simulink model "mchp_acim_dsPIC33A"  (R2025b)
settings: Solver=FixedStepDiscrete  StartTime=0.0  StopTime=25  FixedStep=Ts  RelTol=1e-3  EnableMultiTasking=on
values from neighbouring files (symbols this model uses):
  dataType = 'single'    [mchp_acim_foc_dsPIC33A_data.m]
  PWM_frequency = 20e3    (= 20000)    [mchp_acim_foc_dsPIC33A_data.m]
  PWM_frequency_mc = PWM_frequency    (= 20000)    [mchp_acim_foc_dsPIC33A_data.m]
  SpeedFilterCutoff = 40    [mchp_acim_foc_dsPIC33A_data.m]
  Ts = T_pwm    (= 5e-05)    [mchp_acim_foc_dsPIC33A_data.m]
  Ts_mc = T_pwm_mc    (= 5e-05)    [mchp_acim_foc_dsPIC33A_data.m]
  Ts_motor = T_pwm_mc    (= 5e-05)    [mchp_acim_foc_dsPIC33A_data.m]
  Ts_serialIn = 100e-3    (= 0.1)    [mchp_acim_foc_dsPIC33A_data.m]
undefined symbols (not defined in the file or in its folder): A0, A4, acim, ADC, appState, B0, C10, C11, C6, C7, C8, CS_param, D11, D12, DiscIntNeverNeededParam, estim_pll, estim_qei, inverter, Max, MaxPer, ms, NumBits1, NumBits2, P1, P17, P20, P39, P40, P41, P43, P44, P60, P61, PI_params_SI, Pin, PWM4_Trg1, Resol, s, target, us, VmaxPhase
libraries: simulink x47, MCHP_Blockset x24, mcbcontrolslib x5, mcbeeMathTransformLib x4, slpidlib x4, svdutilitieslib x1, autolibim x1, mcbplantlib x1
(part 1 of 6)
settings Model: ExtModeEnableFloating=off  ExtModeTrigDuration=20  VariantFading=off  Creator=I50990  LastModifiedBy=I73849
settings SolverCC: AlgebraicLoopSolver=TrustRegion
settings OptimizationCC: DefaultParameterBehavior=Inlined  DefaultUnderspecifiedDataType=single  InlineInvariantSignals=on  EnhancedBackFolding=on  BooleansAsBitfields=on  PassReuseOutputArgsAs=Individual arguments  ZeroExternalMemoryAtStartup=off  ZeroInternalMemoryAtStartup=off  OptimizeBlockOrder=speed  DifferentSizesBufferReuse=on  EfficientTunableParamExpr=on
settings DebuggingCC: MultiTaskDSMMsg=none  MultiTaskCondExecSysMsg=none  MultiTaskRateTransMsg=warning  ParameterTunabilityLossMsg=error  ArithmeticOperatorsInVariantConditions=warning
settings HardwareCC: ProdBitPerPointer=32.0  ProdBitPerSizeT=32.0  ProdBitPerPtrDiffT=32.0  ProdLargestAtomicInteger=Long  ProdWordSize=32.0  ProdLongLongMode=on  ProdHWDeviceType=Generic->Custom
settings ModelReferenceCC: ModelReferenceNumInstancesAllowed=Single
settings SFSimCC: MATLABDynamicMemAlloc=off  CustomCodeUndefinedFunction=UseInterfaceOnly
settings RTWCC: SystemTargetFile=MCHP_dsPIC33A_noTMF_stf.tlc  TLCOptions="-aExtModeXCPClassicInterface=0  -aCreateExtModeTypes=1 -aExtModeXCPSimulationTimeInTicks=1"  TemplateMakefile=MCHP_dsPIC33A.tmf  Toolchain=MPLAB XC-DSC - v3.31 for dsPIC DSCs (Microchip)  BuildConfiguration=Specify  GPUComputeCapability=3.5  Description=Microchip Embedded Target dsPIC33A no TMF (real-time)
settings CodeAppCC: ForceParamTrailComments=on  IgnoreCustomStorageClasses=off  MaxIdLength=255.0  OperatorAnnotations=on  SimulinkDataObjDesc=on  SFDataObjDesc=on  InsertBlockDesc=on
settings STFCustomTargetCC: SystemTargetFile=MCHP_dsPIC33A_noTMF_stf.tlc  TargetLangStandard=C99 (ISO)  MultiwordLength=256.0  ConcurrentExecutionCompliant=off  CombineOutputUpdateFcns=on  CombineSignalStateStructs=on  SuppressErrorStatus=on  ERTCustomFileBanners=on  SupportContinuousTime=off  RemoveResetFunc=on  MATLABClassNameForMDSCustomization=Simulink.SoftwareTarget.ERTCustomization  GRTInterface=off  UseToolchainInfoCompliant=on  AssemblyListing=off  LINKER_SCRIPT=p33AK128MC106.gld  OPTIM_GCC=-O2 -mno-eds-warn -mconst-in-data -mlarge-code -mlarge-data -mlarge-scalar -mlarge-aggregate -g -Wa,--reorder  GCC1=xc-dsc-gcc.exe  RTWGenSettings_txt="s.RefMasterBlk='mchp_acim_dsPIC33A/MCHV-230VAC-1.5kW Development Board dsPIC33AK128MC106 MC DIM/Microchip Master';s.ChipIdN='[33  128  106]';s.ChipIdL1='AK';s.ChipIdL2='MC';s.ChipIdL3=' ';s.arch3='33A';s.ChipId='33AK128MC106';s.Arch='8';s.bitFieldsSFR='3';s.ChipRAM='16384';s.ChipRAM_XBegin='16384';s.ChipRAM_dma='[-1 -1]';s.FuseConfigTxt='#pragma config FWDT_WDTEN = SW\\\\n#pragma config FICD_JTAGEN = OFF\\\\n';s.TimeStep_Timer='-1';s.TimeStep_SyncADC='1';s.ADPCFG='0';s.ANSEL_Exist='1';s.ANSEL='[-1 -1 -1 -1 -1 -1 -1 -1 -1 -1 -1]';s.TRIS='[65535  65535  64990  65503     -1     -1     -1     -1     -1     -1     -1     -1     -1     -1     -1     -1     -1     -1     -1     -1     -1     -1     -1     -1     -1     -1     -1     -1     -1     -1     -1     -1     -1     -1     -1     -1     -1     -1     -1     -1     -1     -1     -1     -1     -1     -1     -1     -1     -1     -1     -1     -1     -1     -1     -1     -1     -1]';s.RPOR='[-1         -1         -1         -1         -1         -1         -1         -1         -1         -1     589824         -1         -1         -1  184549376         -1         -1         -1         -1         -1]';s.RPINR='[-1       -1       -1       -1       -1       -1       -1    10279       -1  3997740       -1       -1       -1       -1       -1       -1       -1       -1       -1       -1       -1       -1]';s.LATSET='[-1 -1 -1 -1 -1 -1 -1 -1 -1 -1 -1 -1 -1 -1 -1 -1 -1 -1 -1 -1 -1 -1 -1 -1 -1 -1 -1 -1 -1 -1 -1 -1 -1 -1 -1 -1 -1 -1 -1 -1 -1 -1 -1 -1 -1 -1 -1 -1 -1 -1 -1 -1 -1 -1 -1 -1 -1]';s.LATCLR='[-1 -1 -1 -1 -1 -1 -1 -1 -1 -1 -1 -1 -1 -1 -1 -1 -1 -1 -1 -1 -1 -1 -1 -1 -1 -1 -1 -1 -1 -1 -1 -1 -1 -1 -1 -1 -1 -1 -1 -1 -1 -1 -1 -1 -1 -1 -1 -1 -1 -1 -1 -1 -1 -1 -1 -1 -1]';s.ODC='[-1 -1 -1 -1 -1 -1 -1 -1 -1 -1 -1 -1 -1 -1 -1 -1 -1 -1 -1 -1 -1 -1 -1 -1 -1 -1 -1 -1 -1 -1 -1 -1 -1 -1 -1 -1 -1 -1 -1 -1 -1 -1 -1 -1 -1 -1 -1 -1 -1 -1 -1 -1 -1 -1 -1 -1 -1]';s.CNPU='[-1 -1 -1 -1 -1 -1 -1 -1 -1 -1 -1 -1 -1 -1 -1 -1 -1 -1 -1 -1 -1 -1 -1 -1 -1 -1 -1 -1 -1 -1 -1 -1 -1 -1 -1 -1 -1 -1 -1 -1 -1 -1 -1 -1 -1 -1 -1 -1 -1 -1 -1 -1 -1 -1 -1 -1 -1]';s.CNPD='[-1 -1 -1 -1 -1 -1 -1 -1 -1 -1 -1 -1 -1 -1 -1 -1 -1 -1 -1 -1 -1 -1 -1 -1 -1 -1 -1 -1 -1 -1 -1 -1 -1 -1 -1 -1 -1 -1 -1 -1 -1 -1 -1 -1 -1 -1 -1 -1 -1 -1 -1 -1 -1 -1 -1 -1 -1]';s.PortConfigTxt=' ';s.CLKDIV='0';s.PLLFBD='-1';s.PLLDIV='16815713';s.QUARTZ='8000000';s.SWITCH_OSC='16386';s.PLLRNG='-1';s.MASTER_BusyFlag='-1';s.POWERSAVE='0';s.MIPS='200000000';s.FLASH_ECC='0';s.PBxDIV='[-1]';s.CLKx_INTDIV='[-1 -1 -1 -1  0  1  0  0  0 -1 -1  0 -1]';s.CLKx_FRACDIV='[-1   -1   -1   -1    0  256    0    0    0   -1   -1    0   -1]';s.AN_type2='1';s.ACLKCON_reg='-1';s.nTIMERS='1';s.nSCCP='4';s.DOS_04094_cpu_33a_v1_dspic33a='1';s.DOS_04436_perseus_dspic33a='1';s.DOS_04928_gpio_ports_upb_v2_dspic33a='1';s.DOS_02672_math_progcrc_upb_v1_dspic33a='1';s.DOS_04993_sec_32bit_cp_upb_v1_dspic33a='1';s.DOS_03459_adc_pc_ctrl_upb_v2_dspic33a='1';s.DOS_04302_pwm_pc_upb_v3_dspic33a='1';s.DOS_03076_uart_protocol_upb_v1_dspic33a='1';s.DOS_01482_spi_i2s_upb_v1_dspic33a='1';s.DOS_05155_i2c_upb_v4_dspic33a='1';s.DOS_02359_sent_j2716_upb_v1_dspic33a='1';s.DOS_05177_qei_32b_upb_v2_dspic33a='1';s.DOS_01512_ccp_mccp_upb_v1_dspic33a='1';s.DOS_03496_dac_pdm_nbit_upb_v2_dspic33a='1';s.DOS_02673_tmr_classa_upb_v1_dspic33a='1';s.DOS_04776_perf_mon_upb_v1_dspic33a='1';s.DOS_03680_pfm_pbu_33a_upb_v1_dspic33a='1';s.DOS_04649_sec_pac_upb_v0_dspic33a='1';s.DOS_03966_io_integrity_monitor_upb_v1_dspic33a='1';s.DOS_04641_biss_master_upb_v1_dspic33a='1';s.DOS_04077_dma_upb_v1_dspic33a='1';s.DOS_04549_nvm_ctrl_32bit_upb_v1_dspic33a='1';s.DOS_04449_clk_cru_33a_upb_v1_dspic33a='1';s.DOS_03850_clk_monitor_upb_v1_dspic33a='1';s.DOS_04342_osc_rc8mhz_ctrl_upb_v4_dspic33a='1';s.DOS_04650_wdt_upb_v4_dspic33a='1';s.DOS_05178_ptg_pc_upb_v2_dspic33a='1';s.DOS_04181_data_ram_ctrl_upb_v1_dspic33a='1';s.DOS_04735_wdt_dmt_upb_v6_dspic33a='1';s.DOS_01577_cla_clc_upb_v1_dspic33a='1';s.DOS_03516_pwr_sib_upb_v3_dspic33a='1';s.DOS_03495_amp_pad_opamp_ctrl_upb_v2_dspic33a='1';s.DOS_05830_blueRidge_dspic33a='0';s.DOS_05972_adc_12b_upb_v3_itc_dspic33a='0';s.DOS_05404_adc_pc_ctrl_upb_v3_dspic33a='0';s.DOS_05226_pwm_pc_upb_v4_dspic33a='0';s.DOS_05514_qei_32b_upb_v3_dspic33a='0';s.DOS_05431_dac_pdm_nbit_upb_v3_dspic33a='0';s.DOS_05828_pfm_pbu_33a_upb_v2_dspic33a='0';s.DOS_05765_math_rdc_upb_v1_32bit='0';s.DOS_05908_math_cic_upb_v2_32bit='0';s.DOS_05801_dma_upb_v2_dspic33a='0';s.DOS_05461_pwr_sib_upb_v4_dspic33a='0';s.DOS_05420_amp_vref_ctl_upb_v1_dspic33a='0';s.DOS_05592_pwr_monitor_sib_upb_v1='0';s.DOS_05924_bus_dual_die_upb_v2='0';s.DOS_06048_sec_cam_v3_dspic33a='0';s.DOS_05922_i3c_upb_v1_32bit='0';s.DOS_06006_adc_soft_code_seq_v2_dspic33a='0';s.DOS_05442_icd_trace_33a_v1_dspic33a='0';s.DOS_04537_can_fd_upb_v3_dspic33a='0';s.DOS_05308_pegasus_dspic33a='0';s.DOS_02976_adc_12b_upb_v2_dspic33a='0';s.DOS_05226_apwm_pc_upb_v4_dspic33a='0';s.DOS_04649_sec_pac_upb_v1_dspic33a='0';s.DOS_05346_sec_cam_v2_dspic33a='0';s.DOS_03267_adc_soft_code_seq_v1_dspic33a='0';s.DOS_05557_serpens_dspic33a='0';s.DOS_05972_adc_12b_upb_v3_adc_dspic33a='0';s.DOS_03681_bmx_33a_upb_v1_dspic33a='0';s.DOS_02050_tmr_rtcc_upb_v1_dspic33a='0';s.DOS_04649_sec_pac_upb_serpens_dspic33a='0';s.DOS_05692_pwr_sib_upb_v5_dspic33a='0';s.DOS_06006_adc_soft_code_seq_v2_adc_dspic33a='0';s.DOS_02551_cpu_16bit_v7='0';s.DOS_01520_wdt_dmt_upb_v1_16bit='0';s.DOS_02359a_sent_j2716_upb_v1='0';s.DOS_02672_math_progcrc_upb_v1_16bit='0';s.DOS_01577_cla_clc_upb_v1='0';s.DOS_02915_ecc_v2='0';s.DOS_02673_tmr_classa_upb_v1_16bit='0';s.DOS_01494_qei_32b_upb_v1_16bit='0';s.DOS_02472_ppi_pmp16_upb_v1_16bit='0';s.DOS_01441_i2c_upb_v1_16bit_TLAH='0';s.DOS_03076_uart_protocol_upb_v1_16bit='0';s.DOS_01482='0';s.DOS_01483_pwm_16bit='0';s.DOS_02949_WACG='0';s.DOS_02316_nvm_ctrl_v1_16bit='0';s.DOS_03349_amp_pad_opamp_ctrl_upb_v1='0';s.DOS_02653_afe_current_bias_ctrl_upb_v1_16bit='0';s.DOS_01459_ptg_pc_upb_v1_16bit='0';s.DOS_01512_ccp_mccp_upb_v1_16bit='0';s.DOS_02519_dma_sfr_16bit_v2='0';s.DOS_02508c11='0';s.DOS_02475_dac_pdm_nbit_upb_v1_16bit='0';s.DOS_02467_gpio_upb_v1_16bit='0';s.DOS_00805_rst_integration_v4='0';s.DOS_02659_clk_sib_v12='0';s.DOS_02237_osc_dco_ctrl_upb_v1_16bit='0';s.DOS_02674_wdt_upb_v1_16bit='0';s.DOS_01407='0';s.DOS_03247_CAN_FD_UPB_V2_16_bit='0';s.DOS_03994_WAC07='0';s.DOS_02552_msi_upb_v1_Master='0';s.DOS_03667_pwm_pc_upb_v2_16bit='0';s.DOS_04180_drm_ctrl_ecc_v1='0';s.DOS_03431_STX03='0';s.DOS_03516_pwr_sib_upb_v3='0';s.DOS_02552_msi_upb_v1_Slave='0';s.DOS_04621_amp_pga_ctrl_upb_v3='0';s.DOS_02497_WACV='0';s.DOS_02593_amp_pga_ctrl_pb_v2_16bit='0';s.DOS_01461_afe_ctmu_con_upb_v1_16bit='0';s.DOS_02497_WACA='0';s.DOS_02478_uart_irda_upb_v1_16bit='0';s.DOS_00929='0';s.DOS_01198='0';s.DOS_03029_WACH='0';s.DOS_01483_apwm_16bit='0';s.DOS_04797_WAC0A='0';s.DOS_04884_WAC0B='0';s.DOS_04797_WAC09='0';s.DOS_03662_WACU='0';s.DOS_00794='0';s.DOS_00931='0';s.DOS_00932='0';s.DOS_00942='0';s.DOS_00938='0';s.DOS_00996='0';s.DOS_00997='0';s.DOS_00998='0';s.DOS_00209='0';s.DOS_01555_adc='0';s.DOS_01293='0';s.DOS_00828='0';s.DOS_01116='0';s.DOS_01017_RPORx='0';s.DOS_01017_RPINRx='0';s.DOS_01555_nvm_tsmc18_v2_16bit='0';s.DOS_00804='0';s.DOS_00826='0';s.DOS_01555_TLAK_PMDx='0';s.DOS_01555_TLAK_INT_='0';s.DOS_00933='0';s.DOS_01555='0';s.DOS_01555_ptg='0';s.DOS_00958='0';s.DOS_01117_PORTx='0';s.DOS_00999='0';s.DOS_01041='0';s.DOS_00892='0';s.DOS_01287_TLAC_PMDx='0';s.DOS_01287_TLAC_INT_='0';s.DOS_01424='0';s.DOS_01332='0';s.DOS_01468_PMBA_current_source='0';s.DOS_02291_PGA='0';s.DOS_01467_Comparator='0';s.DOS_01498_TLAY='0';s.DOS_00993_PLL_120MHz='0';s.DOS_01332_ptg_pc_v1='0';s.DOS_00958_pwm_TLAY='0';s.TLAY_IOPorts='0';s.DOS_00929q='0';s.DOS_02415_spi_v5='0';s.DOS_RPINRx_16bit_2='0';s.DOS_01497_TLAH_PMDx='0';s.DOS_02550_TLAL_INT='0';s.DOS_00958_pwm_TLAH='0';s.DOS_01287_TLAH_INT_='0';s.DOS_01113='0';s.DOS_01017_PMDx='0';s.DOS_00927='0';s.DOS_01080='0';s.DOS_00794_cpu_16bit_v3='0';s.DOS_02192_TLCD_PMDx='0';s.DOS_02192_TLCD_INT_='0';s.DOS_02192_cmp='0';s.DOS_00958_pwm_TLCD='0';s.DOS_02192_PORTx_TLCD='0';s.DOS_00936='0';s.DOS_00995='0';s.DOS_00546='0';s.DOS_00474='0';s.DOS_02481_WACP_Config='0';s.DOS_03088_pfm_cache_ocp_v2_WACK='0';s.DOS_02819_pfm_ctrl_32bit_upb_v2='0';s.DOS_02674_wdt_upb_v1_32bit='0';s.DOS_01520_wdt_dmt_upb_v1='0';s.DOS_02869_icd_jtag_bvci_upb_v2='0';s.DOS_02823_WACJ_clk_cru_upb_v2='0';s.DOS_02823_WACN_clk_cru_upb_v2='0';s.DOS_01423_RPINRx='0';s.DOS_02481_RPORx='0';s.DOS_02511_pwr_sib_upb_v1_32bit='0';s.DOS_02907_WACP_int_evic_v3='0';s.DOS_01500_dma_bvci_v2='0';s.DOS_02141_tmr_classa_pb_v2='0';s.DOS_02815_tmr_classb_upb_v1='0';s.DOS_00740_icap_pb_v1='0';s.DOS_00749_ocmp_pb_v1='0';s.DOS_01441_i2c_upb_v1_32bit='0';s.DOS_01329_spi_pb_v2='0';s.DOS_02478_uart_irda_upb_v1_32bit='0';s.DOS_01477_pwm_mc_upb_v1='0';s.DOS_01494_qei_32b_upb_v1='0';s.DOS_03554_cmp_control_upb_v2_32bit='0';s.DOS_01445_dac_nbit__control_upb_v1_32bit='0';s.DOS_01461_afe_ctmu_con_upb_v1='0';s.DOS_01577_cla_clc_upb_v1_32bit='0';s.DOS_02467_gpio_ports_upb_v1='0';s.DOS_02508_WACP_adc_sar_ctrl_upb_v1='0';s.DOS_01261_tmr_rtcc_WACJ_K_N_P_pb_v2='0';s.DOS_EIP_00136_ssx_v1='0';s.DOS_02481_WACK_MC_Config='0';s.DOS_02907_WACN_GP_int_evic_v3='0';s.DOS_02508_adc_sar_ctrl_upb_v1_PIC32MK='0';s.DOS_01261_tmr_rtcc_pb_v2='0';s.DOS_01475_lpwr_deep_sleep_ctrl_v2='0';s.DOS_02907_WACN_MC_int_evic_v3='0';s.DOS_03247_can_fd_upb_v2_pic32mk='0';s.DOS_02907_WACK_MC_int_evic_v3='0';s.DOS_02514_dfm_strl_sst_upb_v1='0';s.DOS_02472_ppi_pmp16_upb_v1='0';s.DOS_02813a_usb_otgcore_pb_v3='0';s.DOS_02481_WACJ_MC_Config='0';s.DOS_02569_pfm_cache_ocp_v1='0';s.DOS_02481_WACJ_MC_int_evic_v3='0';s.DOS_01459_ptg_pc_upb_v1_SIC='0';s.DOS_01427_cmp_control_upb_v1_32bit='0';s.DOS_01152_can_bvci_v1='0';s.DOS_02787_WACD_Config='0';s.DOS_00800_dac_4bit_ctrl_pb_v1='0';s.DOS_01539_icd_jtag_pb_v2='0';s.DOS_02823_clk_cru_upb_v2='0';s.DOS_01423_RPORx='0';s.DOS_02907_WACD_int_evic_v3='0';s.DOS_00734_uart_irda_pb_v1='0';s.DOS_00687_tmr_classa_pb_v1='0';s.DOS_00745_tmr_classb_pb_v1='0';s.DOS_02508_adc_sar_ctrl_upb_v1='0';s.DOS_00866_cmp_control_pb_v2='0';s.DOS_01114_eth_bvci_v1='0';s.DOS_02831_usb_clk_rst_v2='0';s.DOS_01643_pfm_cache_ahb_v2='0';s.DOS_EIP_00206r5_sqi_v2='0';s.DOS_EIP_00124_usb_hs_otgcore_v1='0';s.DOS_EIP_00218_math_rng_ahbs_v2='0';s.DOS_EIP_00109_ebi_v1='0';s.DOS_EIP_00158_crypto_v1='0';s.UART_TX_IMPLEMENTATION='[2  2]';s.UART_RX_IMPLEMENTATION='[2  2]';s.UART_TX_DMACHANNEL='[2  1]';s.UART_HALF_DUPLEX_MODE='[0  0]';s.UART_TX_THREAD_PROTECTION='[9  9]';"  ProduceHexOutput=off  PIC_REF=33AK128MC106  BIN2HEX=xc-dsc-bin2hex  MCHP_MULTITHREAD_COMPILATION=on  LinkWithMaster=off  MCHP_CompiledTime_ModelSampleTimes_Txt=s(1).Value=reshape([5e-05 0],1,2);s(1).Description='Discrete 1';s(1).ColorRGBValue=reshape(MCHP_Fun.Hex2num('[3FF0000000000000 3FD1515151515151 3FCD1D1D1D1D1D1D]'),1,3);s(1).Annotation='D1';s(1).TID=0;s(1).Owner=[];s(1).ComponentSampleTimes=[];s(2).Value=reshape([0.0005 0],1,2);s(2).Description='Discrete 2';s(2).ColorRGBValue=reshape(MCHP_Fun.Hex2num('[3FCD1D1D1D1D1D1D 3FE9191919191919 3FC8989898989899]'),1,3);s(2).Annotation='D2';s(2).TID=1;s(2).Owner=[];s(2).ComponentSampleTimes=[];s(3).Value=reshape([0.001 0],1,2);s(3).Description='Discrete 3';s(3).ColorRGBValue=reshape(MCHP_Fun.Hex2num('[3FAC1C1C1C1C1C1C 0000000000000000 3FF0000000000000]'),1,3);s(3).Annotation='D3';s(3).TID=2;s(3).Owner=[];s(3).ComponentSampleTimes=[];s(4).Value=reshape([0.1 0],1,2);s(4).Description='Discrete 4';s(4).ColorRGBValue=reshape(MCHP_Fun.Hex2num('[3FAC1C1C1C1C1C1C 0000000000000000 3FF0000000000000]'),1,3);s(4).Annotation='D4';s(4).TID=3;s(4).Owner=[];s(4).ComponentSampleTimes=[];s(5).Value=reshape([0.5 0],1,2);s(5).Description='Discrete 5';s(5).ColorRGBValue=reshape(MCHP_Fun.Hex2num('[3FAC1C1C1C1C1C1C 0000000000000000 3FF0000000000000]'),1,3);s(5).Annotation='D5';s(5).TID=4;s(5).Owner=[];s(5).ComponentSampleTimes=[];s(6).Value=reshape([Inf Inf],1,2);s(6).Description='Constant';s(6).ColorRGBValue=reshape(MCHP_Fun.Hex2num('[3FEA3A3A3A3A3A3A 3F90101010101010 3FE1717171717171]'),1,3);s(6).Annotation='Inf';s(6).TID=-2;s(6).Owner=[];s(6).ComponentSampleTimes=[];s(7).Value='Source: D1';s(7).Description='Triggered';s(7).ColorRGBValue=reshape(MCHP_Fun.Hex2num('[3FF0000000000000 3FD1515151515151 3FCD1D1D1D1D1D1D]'),1,3);s(7).Annotation='D1';s(7).TID=7;s(7).Owner=[];s(7).ComponentSampleTimes=[];s(8).Value='Source: D4';s(8).Description='Triggered';s(8).ColorRGBValue=reshape(MCHP_Fun.Hex2num('[3FAC1C1C1C1C1C1C 0000000000000000 3FF0000000000000]'),1,3);s(8).Annotation='D4';s(8).TID=8;s(8).Owner=[];s(8).ComponentSampleTimes=[];s(9).Value=[];s(9).Description='Multirate';s(9).ColorRGBValue=reshape(MCHP_Fun.Hex2num('[3FE1717171717171 3FD999999999999A 3F98181818181818]'),1,3);s(9).Annotation='M';s(9).TID=[];s(9).Owner=[];s(9).ComponentSampleTimes=[];  TIMER_PRESCALER="[-1  0 -1 -1 -1]"  HOST_PLATFORM=PC  MCHP_XCP_MemoryBlockParameters=[-1 8]  LDFLAGS='--report-mem,-Map=$(PRODUCT_NAME).map,-cref,-lq-dsp,--memorysummary,memoryfile.xml'  TIMER_START="[0  0]"  TIMER_PERIOD="[0  65535]"  OBJDUMP=xc-dsc-objdump  AR1=xc-dsc-ar  MCHP_AUTO_FLASH=on  GCCPATH=C:/PROGRA~1/MICROC~1/xc-dsc/v3.31/bin  EXTMODE_DATA_UPLOAD=on
settings ERTTargetCC: ExtModeTransport=1.0  ExtModeStaticAlloc=on  ExtModeMaxTrigDuration=20.0  ExtModeStaticAllocSize=4096.0  ExtModeMexFile=ext_xcp  ExtModeMexArgs=1 5 1000000 './mchp_acim_dsPIC33A.X/mchp_acim_dsPIC33A.elf'  ExtModeIntrfLevel=Level2 - Open  ERTSrcFileBannerTemplate=MCHP_dsPIC_code_template.cgt  ERTHdrFileBannerTemplate=MCHP_dsPIC_code_template.cgt  ERTDataSrcFileTemplate=MCHP_dsPIC_code_template.cgt  ERTDataHdrFileTemplate=MCHP_dsPIC_code_template.cgt  ERTCustomFileTemplate=MCHP_main.tlc  MaxLineWidth=110.0  TargetLangStandard=C99 (ISO)  ParMdlRefBuildCompliant=off  CompOptLevelCompliant=off  ConcurrentExecutionCompliant=off  CombineSignalStateStructs=on  SuppressErrorStatus=on  SupportNonInlinedSFcns=on  ModelStepFunctionPrototypeControlCompliant=off  CPPClassGenCompliant=off

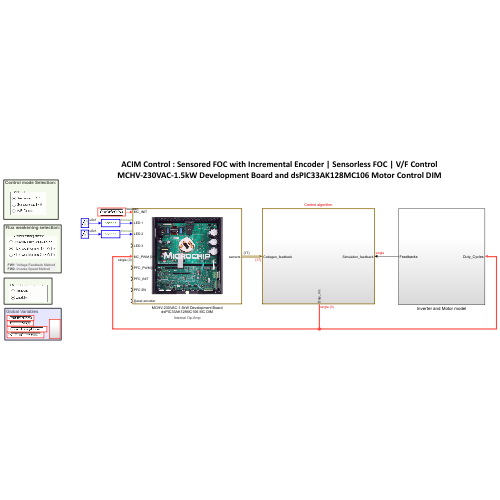
[thumbnail: Simulink's stored preview of the top-level diagram]
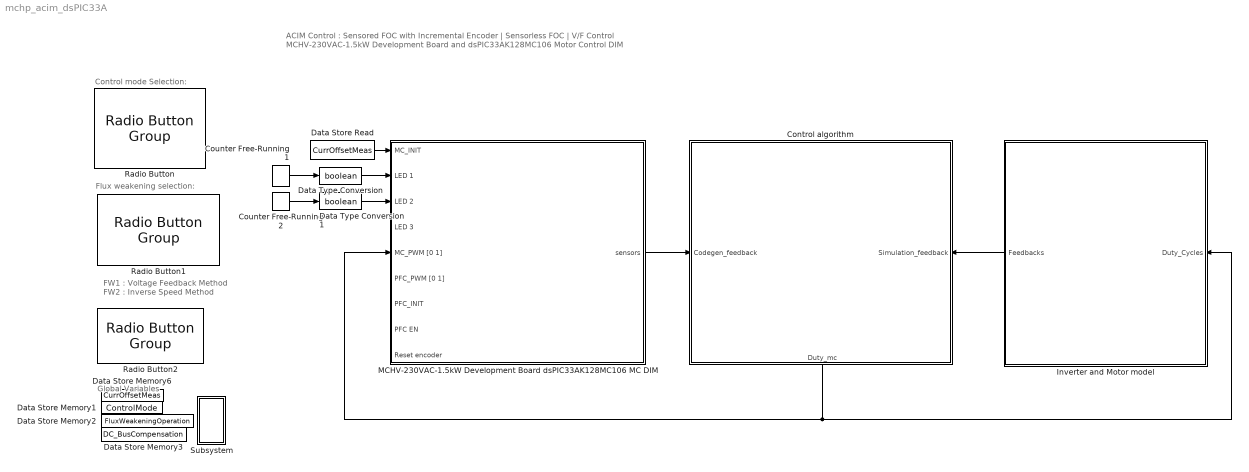
== system mchp_acim_dsPIC33A ==
  note: Flux weakening selection:
  note: Control mode Selection:
  note: FW1 : Voltage Feedback Method
      | FW2 : Inverse Speed Method
  note: ACIM Control : Sensored FOC with Incremental Encoder | Sensorless FOC | V/F Control
      | MCHV-230VAC-1.5kW Development Board and dsPIC33AK128MC106 Motor Control DIM
  note: Global Variables
  Control algorithm : Subsystem
      settings: PortSchema="{\"entries\":[{\"content\":{\"sides\":[{\"content\":{\"connectorIds\":[\"In1\"]},\"type\":\"ConnectorPlacement.EquallySpacedRectSide\",\"uuid\":\"c89745de-36f0-4b44-b5cd-d26457eee3e2\"},{\"content\":{\"connectorIds\":[\"In2\"],\"side\":\"RIGHT\"},\"type\":\"ConnectorPlacement.EquallySpacedRectSide\",\"uuid\":\"ba0a3657-2aaf-4106-ae21-dd806e372604\"},{\"content\":{\"side\":\"TOP\"},\"type\":\"ConnectorPlacement.EquallySpacedRectSide\",\"uuid\":\"08922b73-d2c6-4004-a015-ef2d01c5c594\"},{\"content\":{\"connectorIds\":[\"Out1\"],\"side\":\"BOTTOM\"},\"type\":\"ConnectorPlacement.EquallySpacedRectSide\",\"uuid\":\"8dac9f4c-a0f6-47fa-8215-e4ef0296adee\"}]},\"type\":\"ConnectorPlacement.EquallySpacedConnector\",\"uuid\":\"6afb6d73-dba8-47c2-96c1-0e4670ec24e5\"}],\"packageUris\":[\"http://schema.mathworks.com/mf0/Connector/R2020b\"],\"version\":\"1.0\"}"
  Counter Free-Running1 : simulink/Sources/Counter Free-Running  NumBits=1  tsamp=0.5
  Counter Free-Running2 : simulink/Sources/Counter Free-Running  NumBits=1  tsamp=0.1
  Data Store Memory1 : DataStoreMemory  DataStoreName=ControlMode  ShowAdditionalParam=off  OutDataTypeStr=single
  Data Store Memory2 : DataStoreMemory  DataStoreName=FluxWeakeningOperation  ShowAdditionalParam=off  OutDataTypeStr=single
  Data Store Memory3 : DataStoreMemory  DataStoreName=DC_BusCompensation  ShowAdditionalParam=off  OutDataTypeStr=single
  Data Store Memory6 : DataStoreMemory  DataStoreName=CurrOffsetMeas  ShowAdditionalParam=off  OutDataTypeStr=boolean
  Data Store Read : DataStoreRead  DataStoreName=CurrOffsetMeas  IndexOptions=Index vector (dialog)  Indices=1  OutputSizes=1
  Data Type Conversion : DataTypeConversion  OutDataTypeStr=boolean  SaturateOnIntegerOverflow=off  RndMeth=Floor
  Data Type Conversion1 : DataTypeConversion  OutDataTypeStr=boolean  SaturateOnIntegerOverflow=off  RndMeth=Floor
  Inverter and Motor model : Subsystem
      settings: PortSchema="{\"entries\":[{\"content\":{\"sides\":[{\"content\":{\"connectorIds\":[\"Out1\"]},\"type\":\"ConnectorPlacement.EquallySpacedRectSide\",\"uuid\":\"0f090452-5fb7-46df-a950-ea9694b1cead\"},{\"content\":{\"connectorIds\":[\"In1\"],\"side\":\"RIGHT\"},\"type\":\"ConnectorPlacement.EquallySpacedRectSide\",\"uuid\":\"b5da8933-6809-4c78-9804-1c3e1782adf7\"},{\"content\":{\"side\":\"TOP\"},\"type\":\"ConnectorPlacement.EquallySpacedRectSide\",\"uuid\":\"fa8fe658-a3dd-43aa-a6dc-3e0fc279e57d\"},{\"content\":{\"side\":\"BOTTOM\"},\"type\":\"ConnectorPlacement.EquallySpacedRectSide\",\"uuid\":\"eb8a9e0e-c3b4-4625-a224-3da5ff4020ab\"}]},\"type\":\"ConnectorPlacement.EquallySpacedConnector\",\"uuid\":\"596b008b-4d6c-49a9-9331-e194c409647a\"}],\"packageUris\":[\"http://schema.mathworks.com/mf0/Connector/R2020b\"],\"version\":\"1.0\"}"
  MCHV-230VAC-1.5kW Development Board dsPIC33AK128MC106 MC DIM : Subsystem  mask(MCHV-230VAC-1.5kW - dsPIC33AK128MC106 MC DIM){boardVariants=Internal Op-Amp, n=acim.p, QEIResolution=acim.QEPSlits*4, Switching_Frequency=PWM_frequency, Switching_Frequency_MC=PWM_frequency_mc, DeadTime=inverter.deadtime, QEI_Reset=on logical input (software), QEI_Offset_settings=0, QEIOffset=0}
      mask prompts: boardVariants "Board Variants"; n "Motor Pole Pairs"; QEIResolution "Optical Encoder Resolution Per Mechanical Rotation (lines)"; Switching_Frequency "PFC PWM Switching Frequency (Hz)"; Switching_Frequency_MC "MC PWM Switching Frequency (Hz)"; DeadTime "Dead Time (s)"; QEI_Reset "Optical encoder reset"; QEI_Offset_settings "Optical encoder offset (mechanical in rad)"; QEIOffset "Optical encoder offset (mechanical in rad)"
      mask help:
      | Template for MCHV-230VAC-1.5kW motor control development board with the dsPIC33AK128MC106 Motor Control DIM.
      |
      | Block bus output provices:
      |   - ADC: PFC Inductor current (iL),Input AC Voltage (Vac),Motor Phase currents (Ia, Ib), DC bus voltage and Potentiometer
      |   - Buttons
      |   - QEI position
      |
      | Block inputs:
      |   - MC_INIT to trigger the offset measurement and correction of Ia and Ib
      |   - PFC_INIT to trigger the offset measurement of iL
      |   - LEDs
      |   - Normalized PWM duty cycle value for motor control and PFC
      |
      | NOTE :
      | The system provides two preconfigured PWM switching frequencies: 64 kHz and 16 kHz.
      |
      | The Power Factor Correction (PFC) board is specifically designed to operate at a switching frequency of 64 kHz.
      |
      | When the PFC is enabled, the Motor Control (MC) PWM frequency must be set to 16 kHz to ensure proper synchronization and system performance.
      |
      | If the PFC is disabled, the MC PWM frequency can be set to any value as required by the application.
      |
      | If the PFC is disabled, please ensure that the inputs to PFC_PWM, PFC_EN, and PFC_INIT are set to zero.
      mask init:
      | BlksQEI = find_system(gcb,'FollowLinks','on','LookUnderMasks','all','ReferenceBlock','MCHP_Blockset/QEI/QEI');
      | QEI_Reset = get_param(gcb,'QEI_Reset');
      | if numel(BlksQEI) >= 1
      |     switch QEI_Reset
      |         case 'on index signal'
      |             set_param(BlksQEI{1},'PIMOD_mode','RESET position on each INDEX event');
      |         case 'on logical input (software)'        
      |             set_param(BlksQEI{1},'PIMOD_mode','position is cyclique between user defined boundaries'); 
      |         case 'custom setting'
      |             % do nothing 
      |     end
      | end % if
      | 
      |     BlksOpAmp = find_system(gcb,'FollowLinks','on','IncludeCommented','on','LookUnderMasks','all','ReferenceBlock','MCHP_Blockset/Analog IO/Op-Amp');
      |     if numel(BlksOpAmp) >= 1
      |         boardVariants = get_param(gcb,'boardVariants');
      |         switch boardVariants
      |             case 'Internal Op-Amp'
      |                 set_param(BlksOpAmp{1},'Commented','off');
      |             case 'External Op-Amp'
      |                 set_param(BlksOpAmp{1},'Commented','on');
      |         end
      |     end % if
      settings: AttributesFormatString=%<boardVariants>
      mask Help: https://forum.microchip.com/s/sub-forums?&subForumId=a553l000000J2rNAAS&forumId=a553l000000J2pvAAC&subForumName=MATLAB&forumName=Development%20Tools&page=1&offset=0
      mask TypeOptions boardVariants: Internal Op-Amp | External Op-Amp
      mask TypeOptions QEI_Reset: on index signal | on logical input (software) | custom setting
      mask Callback QEI_Reset:
      | QEI_Reset = get_param(gcb,'QEI_Reset');
      | switch QEI_Reset
      |     case 'on index signal'
      |         QEIOffset = MCHP_Fun.Evalin('base','QEIOffset');
      |         set_param(gcb,'QEIOffset',num2str(QEIOffset));
      |         set_param(gcb,'MaskVisibilities',{'on';'on';'on';'on';'on';'on';'on';'off';'on'});
      |     case 'on logical input (software)'
      |         set_param(gcb,'QEIOffset','0');
      |         set_param(gcb,'MaskVisibilities',{'on';'on';'on';'on';'on';'on';'on';'off';'off'});
      |     case 'custom setting'
      |         set_param(gcb,'MaskVisibilities',{'on';'on';'on';'on';'on';'on';'on';'off';'on'});
      |         % do nothing
      | end
      mask DialogControl boardParameters Prompt: Board
      mask DialogControl MotorParameters Prompt: Motor
      mask DialogControl n Tooltip: Number of pole pairs of the motor
      mask DialogControl QEIResolution Tooltip: encoder resolution per mechanical rotation
      mask DialogControl PWMParameters Prompt: PWM
      mask DialogControl QEIParameters Prompt: QEI
      mask DialogControl QEI_Reset Tooltip: enable encoder index signal if available. Otherwise align motor by applying a tension and set the rst input to 1
      mask DialogControl QEI_Offset_settings Tooltip: offset angle between encoder index and motor winding reference axis applied on theta_m and theta_e
      mask Display: image('MCHV_230VAC_1.5kW_new.png');
  Radio Button : RadioButtonGroup  LabelPosition=Hide  SelectedLabel=Sensored FOC  ButtonGroupName=Control mode
  Radio Button1 : RadioButtonGroup  LabelPosition=Hide  SelectedLabel=Flux weakening 1 (FW1))  ButtonGroupName=Flux weakening mode
  Radio Button2 : RadioButtonGroup  LabelPosition=Hide  SelectedLabel=Enable  ButtonGroupName=DC bus compensation
  Subsystem : Subsystem
  wires:
  Data Type Conversion1/1 -> MCHV-230VAC-1.5kW Development Board dsPIC33AK128MC106 MC DIM/3(LED 2)
  Counter Free-Running1/1 -> Data Type Conversion/1
  Counter Free-Running2/1 -> Data Type Conversion1/1
  MCHV-230VAC-1.5kW Development Board dsPIC33AK128MC106 MC DIM/1(sensors) -> Control algorithm/1(Codegen_feedback)
  Data Type Conversion/1 -> MCHV-230VAC-1.5kW Development Board dsPIC33AK128MC106 MC DIM/2(LED 1)
  Data Store Read/1 -> MCHV-230VAC-1.5kW Development Board dsPIC33AK128MC106 MC DIM/1(MC_INIT)
  Inverter and Motor model/1(Feedbacks) -> Control algorithm/2(Simulation_feedback)
  Control algorithm/1(Duty_mc) -> Inverter and Motor model/1(Duty_Cycles), MCHV-230VAC-1.5kW Development Board dsPIC33AK128MC106 MC DIM/5(MC_PWM [0 1])

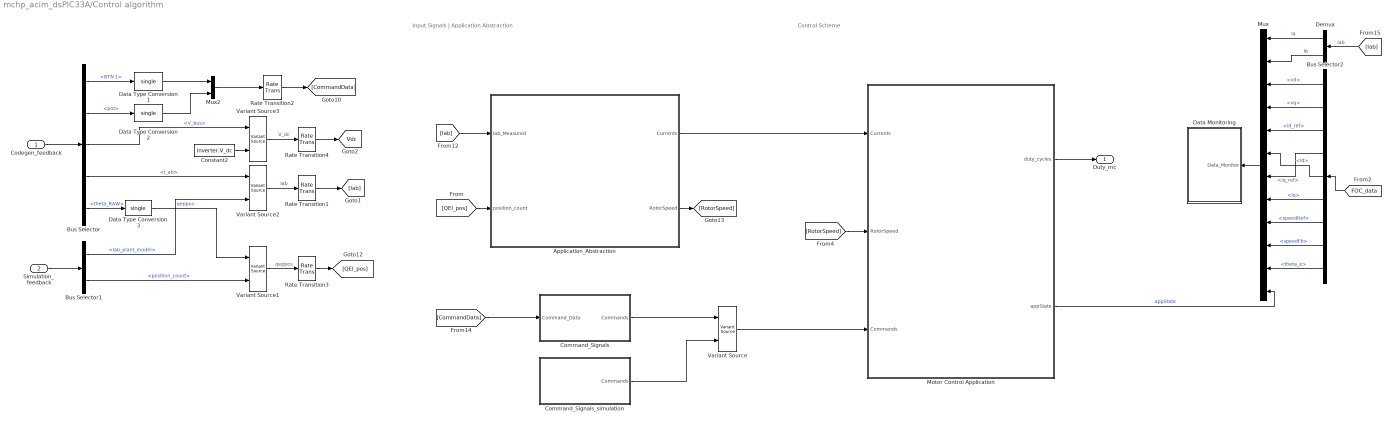
== system mchp_acim_dsPIC33A/Control algorithm ==
  note: Input Signals | Application Abstraction
  note: Control Scheme
  Codegen_feedback : Inport
  Simulation_feedback : Inport  Port=2
  Application_Abstraction : Subsystem
  Bus Selector : BusSelector  OutputSignals=BTN.BTN 1,ADC.pot,ADC.V_bus,ADC.I_ab,optical coder.RAW.theta_RAW
  Bus Selector1 : BusSelector  OutputSignals=Iab_plant_model,position_count
  Bus Selector2 : BusSelector  OutputSignals=vd,vq,id_ref,iq_ref,Id,Iq,speedRef,speedFb,theta_e
  Command_Signals : Subsystem
  Command_Signals_simulation : Subsystem
  Constant2 : Constant  Value=inverter.V_dc  OutDataTypeStr=single
  Data Monitoring : Subsystem
  Data Type Conversion1 : DataTypeConversion  OutDataTypeStr=single  SaturateOnIntegerOverflow=off  RndMeth=Floor
  Data Type Conversion2 : DataTypeConversion  OutDataTypeStr=single  SaturateOnIntegerOverflow=off  RndMeth=Floor
  Data Type Conversion3 : DataTypeConversion  OutDataTypeStr=single  SaturateOnIntegerOverflow=off  RndMeth=Floor
  Demux : Demux  Outputs=2
  Motor Control Application : Subsystem
  Mux : Mux  Inputs=12
  Mux2 : Mux  Inputs=2
  Rate Transition{1..4} (4 alike) : RateTransition  OutPortSampleTime=Ts_mc
  Variant Source{,1..3} (4 alike) : VariantSource  VariantControlMode=sim codegen switching  VariantControls={(codegen), (sim)}
  Duty_mc : Outport
  tag scope: Vdc=global
  wires:
  Codegen_feedback/1 -> Bus Selector/1
  Demux/1 -> Mux/1  "Ia"
  Application_Abstraction/1(Currents) -> Motor Control Application/1(Currents)
  [CommandData] -> Command_Signals/1(Command_Data)
  [Iab] -> Application_Abstraction/1(Iab_Measured)
  Variant Source/1 -> Motor Control Application/3(Commands)
  Motor Control Application/1(duty_cycles) -> Duty_mc/1
  Bus Selector/2 -> Data Type Conversion2/1  "<pot>"
  Mux2/1 -> Rate Transition2/1
  Data Type Conversion2/1 -> Mux2/2
  Data Type Conversion1/1 -> Mux2/1
  Bus Selector/1 -> Data Type Conversion1/1  "<BTN 1>"
  Bus Selector/4 -> Variant Source2/1  "<I_ab>"
  Mux/1 -> Data Monitoring/1(Data_Monitor)
  [Iab] -> Demux/1  "Iab"
  Application_Abstraction/2(RotorSpeed) -> [RotorSpeed]
  [RotorSpeed] -> Motor Control Application/2(RotorSpeed)
  Demux/2 -> Mux/2  "Ib"
  [QEI_pos] -> Application_Abstraction/2(position_count)
  Variant Source1/1 -> Rate Transition3/1  "qeppos"
  Command_Signals_simulation/1(Commands) -> Variant Source/2
  Command_Signals/1(Commands) -> Variant Source/1
  Variant Source2/1 -> Rate Transition1/1  "Iab"
  Data Type Conversion3/1 -> Variant Source1/1  "qeppos"
  Simulation_feedback/1 -> Bus Selector1/1
  Bus Selector1/1 -> Variant Source2/2  "<Iab_plant_model>"
  Bus Selector1/2 -> Variant Source1/2  "<position_count>"
  Bus Selector/3 -> Variant Source3/1  "<V_bus>"
  Rate Transition3/1 -> [QEI_pos]
  Rate Transition1/1 -> [Iab]
  Rate Transition2/1 -> [CommandData]
  [FOC_data] -> Bus Selector2/1
  Bus Selector2/2 -> Mux/4  "<vq>"
  Bus Selector2/1 -> Mux/3  "<vd>"
  Bus Selector2/4 -> Mux/7  "<iq_ref>"
  Bus Selector2/3 -> Mux/5  "<id_ref>"
  Bus Selector2/5 -> Mux/6  "<Id>"
  Bus Selector2/6 -> Mux/8  "<Iq>"
  Bus Selector2/8 -> Mux/10  "<speedFb>"
  Bus Selector2/7 -> Mux/9  "<speedRef>"
  Motor Control Application/2(appState) -> Mux/12  "appState"
  Variant Source3/1 -> Rate Transition4/1  "V_dc"
  Constant2/1 -> Variant Source3/2
  Rate Transition4/1 -> [Vdc]
  Bus Selector/5 -> Data Type Conversion3/1  "<theta_RAW>"
  Bus Selector2/9 -> Mux/11  "<theta_e>"

== system mchp_acim_dsPIC33A/Inverter and Motor model ==
  Duty_Cycles : Inport
  Codegeneration : Subsystem
  Simulation : Subsystem
  Variant Sink : VariantSink  VariantControlMode=sim codegen switching  VariantControls={(codegen), (sim)}
  Variant Source : VariantSource  VariantControlMode=sim codegen switching  VariantControls={(codegen), (sim)}
  Feedbacks : Outport  VectorParamsAs1DForOutWhenUnconnected=off
  wires:
  Simulation/1(Feedbacks) -> Variant Source/2
  Duty_Cycles/1 -> Variant Sink/1
  Variant Sink/2 -> Simulation/1(Duty_Cycles)
  Variant Sink/1 -> Codegeneration/1(Duty_Cycles)
  Codegeneration/1(Feedbacks) -> Variant Source/1
  Variant Source/1 -> Feedbacks/1
